simulink model "navigation_degine"  (R2022b)
settings: Solver=ode4  StartTime=TIME.start  StopTime=TIME.final  FixedStep=TIME.sampling  RelTol=1e-3
values from neighbouring files (symbols this model uses):
  Cb2n_init = dcm(bf_euler_true(1, ENUM.PHI),                 bf_euler_true(1, ENUM.THE),                 bf_euler_true(1, ENUM.PSI))'    [HW2_navigation_degine.m]
  EARTH = struct('Re',  6378137,                'Rm',  0.,                'Rp',  0.,                'We',  7.292115e-5,                 'g0',  9.780318,                'e2',  6.6943799014e-3)    [HW2_navigation_degine.m]
libraries: matrix_library x1
settings Model: Creator=jarry_goon  LastModifiedBy=jarry_goon

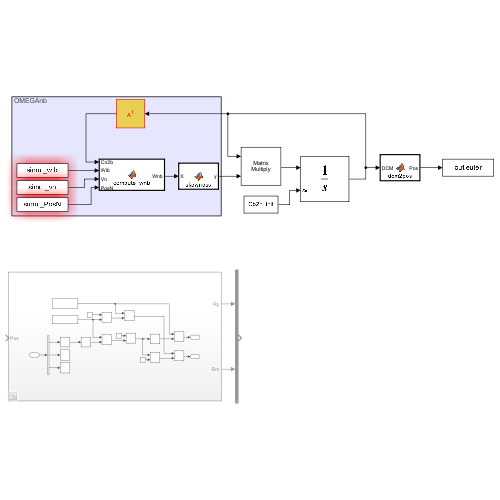
[thumbnail: Simulink's stored preview of the top-level diagram]
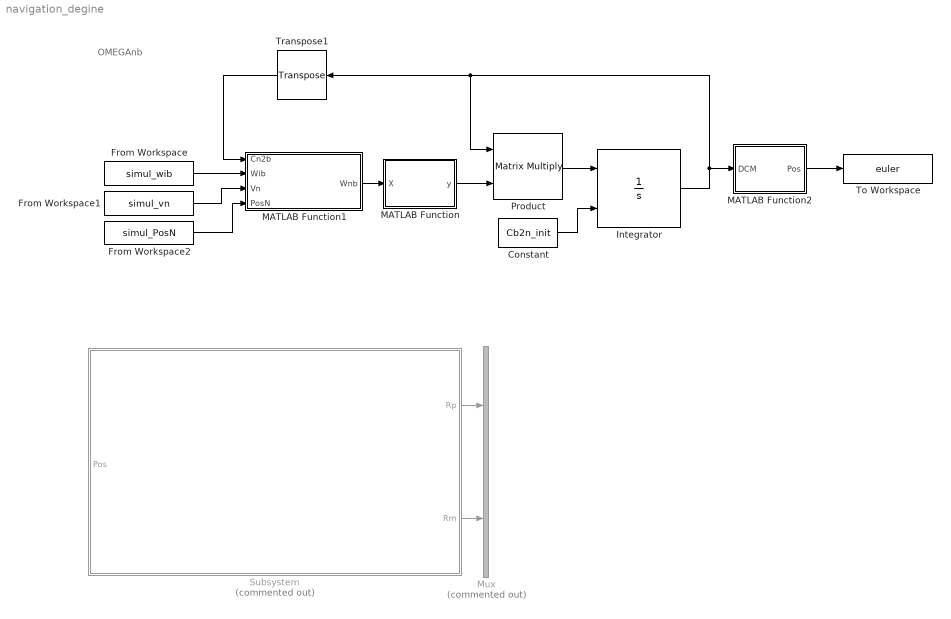
== system navigation_degine ==
  note: OMEGAnb
  Constant : Constant  Value=Cb2n_init
  From Workspace : FromWorkspace  VariableName=simul_wib  OutputAfterFinalValue=Holding final value
  From Workspace1 : FromWorkspace  VariableName=simul_vn  OutputAfterFinalValue=Holding final value
  From Workspace2 : FromWorkspace  VariableName=simul_PosN  OutputAfterFinalValue=Holding final value
  Integrator : Integrator  InitialConditionSource=external  InitialCondition=Cb2n_init
  MATLAB Function : MATLAB Function  TreatAsAtomicUnit=on
  MATLAB Function1 : MATLAB Function  TreatAsAtomicUnit=on
  MATLAB Function2 : MATLAB Function  TreatAsAtomicUnit=on
  Mux : Mux  Commented=on  Inputs=2
  Product : Product  Multiplication=Matrix(*)
  Subsystem : Subsystem  Commented=on
  To Workspace : ToWorkspace  VariableName=euler  SampleTime=-1
      settings: Save2DSignal=2-D array (concatenate along first dimension)
  Transpose1 : matrix_library/Transpose
  wires:
  MATLAB Function1/1(Wnb) -> MATLAB Function/1(X)
  MATLAB Function/1(y) -> Product/2
  Integrator/1 -> Product/1, Transpose1/1, MATLAB Function2/1(DCM)
  MATLAB Function2/1(Pos) -> To Workspace/1
  From Workspace/1 -> MATLAB Function1/2(Wib)
  From Workspace1/1 -> MATLAB Function1/3(Vn)
  Transpose1/1 -> MATLAB Function1/1(Cn2b)
  From Workspace2/1 -> MATLAB Function1/4(PosN)
  Product/1 -> Integrator/1
  Subsystem/1(Rp) -> Mux/1
  Subsystem/2(Rm) -> Mux/2
  Constant/1 -> Integrator/2

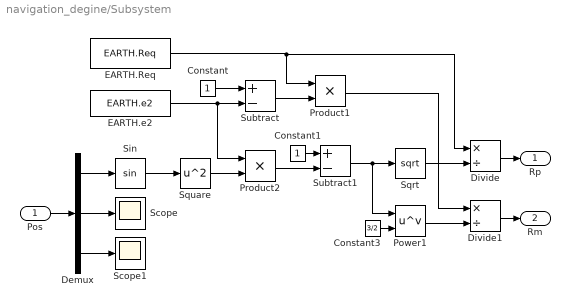
== system navigation_degine/Subsystem ==
  Pos : Inport
  Constant : Constant
  Constant1 : Constant
  Constant3 : Constant  Value=3/2
  Demux : Demux  Outputs=3
  Divide : Product  Inputs=*/
  Divide1 : Product  Inputs=*/
  EARTH.Req : Constant  Value=EARTH.Req
  EARTH.e2 : Constant  Value=EARTH.e2
  Power1 : Math  Operator=pow
  Product1 : Product
  Product2 : Product
  Scope : Scope
  Scope1 : Scope
  Sin : Trigonometry
  Sqrt : Sqrt
  Square : Math  Operator=square
  Subtract : Sum  Inputs=+-
  Subtract1 : Sum  Inputs=+-
  Rp : Outport
  Rm : Outport  Port=2
  wires:
  Constant1/1 -> Subtract1/1
  Demux/1 -> Sin/1
  Power1/1 -> Divide1/2
  Subtract1/1 -> Power1/1, Sqrt/1
  Constant/1 -> Subtract/1
  Sqrt/1 -> Divide/2
  EARTH.Req/1 -> Divide/1, Product1/1
  Sin/1 -> Square/1
  Subtract/1 -> Product1/2
  Divide1/1 -> Rm/1
  Product1/1 -> Divide1/1
  Pos/1 -> Demux/1
  Product2/1 -> Subtract1/2
  EARTH.e2/1 -> Product2/1, Subtract/2
  Constant3/1 -> Power1/2
  Square/1 -> Product2/2
  Divide/1 -> Rp/1
  Demux/2 -> Scope/1
  Demux/3 -> Scope1/1

== matlab function navigation_degine/MATLAB Function1 ==
  data: Cn2b input; Wnb output; Wib input; Vn input; PosN input
function Wnb = compute_wnb(Cn2b, Wib, Vn, PosN)
%COMPUTE_WNB
%   자세한 설명 위치
arguments
    Cn2b (3, 3) double
    Wib (1, 3) double
    Vn (1, 3) double
    PosN (1, 3) double
end

Re = 6478137;
e2 = 6.6943799014e-3;
We = 7.292115e-5;

L = PosN(1);
h = PosN(3);

Rm = Re * (1 - e2) / (1 - e2 * sin(L)^2)^(3/2);
Rp = Re / sqrt(1 - e2 * sin(L)^2);

nav_wen = [Vn(2) / (Rp + h);
          -Vn(1) / (Rm + h);
          -Vn(2) * tan(L) / (Rm + h)];

nav_wie = [cos(L) * We;
           0;
          -sin(L) * We];

nav_win = Cn2b * (nav_wie + nav_wen);

Wnb = Wib' - nav_win;

end

== matlab function navigation_degine/MATLAB Function ==
  data: X input; y output
function y = skewness(X)
%SKEWNESS 입력된 벡터로 왜대칭행렬(Skew-symmetric Matrix)를 만듭니다.
%   

arguments
    X (3, 1) double
end

y = [0     -X(3)   X(2);
     X(3)   0     -X(1);
    -X(2)   X(1)   0];

end

== matlab function navigation_degine/MATLAB Function2 ==
  data: DCM input; Pos output
function Pos = dcm2pos(DCM)
%DCM2POS 이 함수의 요약 설명 위치
%   자세한 설명 위치
arguments
    DCM (3, 3) double
end

psi = atan2(DCM(2, 1), DCM(1, 1));
theta = asin(-DCM(3, 1));
phi = atan2(DCM(3, 2), DCM(3, 3));

Pos = [phi, theta, psi];
end
